simulink model "IADC_wi_SarGainError"  (Simulink 10.0)
settings: Solver=ode45  StartTime=0.0  StopTime=100e-6  RelTol=1e-3  EnableMultiTasking=on
values from neighbouring files (symbols this model uses):
  A = opgain(i)    [ExCount_wi_OPGainError_cal_m.m]    (also in ExCount_wi_OPGainError_m.m = 10000; ExCount_wi_SarGainError_cal_m.m; ExCount_wi_SarGainError_m.m; IADC_pSNDR_vs_Gain_m.m = opgain(i_opgain))
  a1 = 1/1    (= 1)    [ExCount_wi_OPGainError_cal_m.m]    (also in ExCount_wi_OPGainError_m.m; ExCount_wi_SarGainError_cal_m.m; ExCount_wi_SarGainError_m.m; IADC_pSNDR_vs_Gain_m.m)
  a11 = 1/4    (= 0.25)    [ExCount_wi_OPGainError_cal_m.m]    (also in ExCount_wi_OPGainError_m.m = 1; ExCount_wi_SarGainError_cal_m.m = 1; ExCount_wi_SarGainError_m.m = 1; IADC_pSNDR_vs_Gain_m.m = 1)
  a12 = 1    [ExCount_wi_OPGainError_cal_m.m]    (also in ExCount_wi_OPGainError_m.m; ExCount_wi_SarGainError_cal_m.m; ExCount_wi_SarGainError_m.m; IADC_pSNDR_vs_Gain_m.m)
  a2 = 1/1    (= 1)    [ExCount_wi_OPGainError_cal_m.m]    (also in ExCount_wi_OPGainError_m.m; ExCount_wi_SarGainError_cal_m.m; ExCount_wi_SarGainError_m.m; IADC_pSNDR_vs_Gain_m.m)
  A_binary = opgain_binary(i)    [ExCount_wi_OPGainError_cal_m.m]
  adder_max = vref*1    (= 0.9)    [ExCount_wi_OPGainError_cal_m.m]    (also in ExCount_wi_OPGainError_m.m; ExCount_wi_SarGainError_cal_m.m; ExCount_wi_SarGainError_m.m; IADC_pSNDR_vs_Gain_m.m)
  Amax = vref*1    (= 0.9)    [ExCount_wi_OPGainError_cal_m.m]    (also in ExCount_wi_OPGainError_m.m = 0.45; ExCount_wi_SarGainError_cal_m.m; ExCount_wi_SarGainError_m.m; IADC_pSNDR_vs_Gain_m.m = 0.45)
  b11 = 4/1    (= 4)    [ExCount_wi_OPGainError_cal_m.m]    (also in ExCount_wi_OPGainError_m.m = 1; ExCount_wi_SarGainError_cal_m.m = 1; ExCount_wi_SarGainError_m.m = 1; IADC_pSNDR_vs_Gain_m.m = 1)
  err_dac = 1.051/1000*0    (= 0)    [ExCount_wi_OPGainError_cal_m.m]
  fsig = 21.0e3    (= 21000)    [ExCount_wi_OPGainError_cal_m.m]    (also in ExCount_wi_OPGainError_m.m = 43000; ExCount_wi_SarGainError_cal_m.m; ExCount_wi_SarGainError_m.m; IADC_pSNDR_vs_Gain_m.m = 43000)
  k1 = 1/1    (= 1)    [ExCount_wi_OPGainError_cal_m.m]    (also in ExCount_wi_OPGainError_m.m; ExCount_wi_SarGainError_cal_m.m; ExCount_wi_SarGainError_m.m; IADC_pSNDR_vs_Gain_m.m)
  M = OSR-1    (= 15)    [ExCount_wi_OPGainError_cal_m.m]    (also in ExCount_wi_OPGainError_m.m; ExCount_wi_SarGainError_cal_m.m = 16; ExCount_wi_SarGainError_m.m = 16; IADC_pSNDR_vs_Gain_m.m)
  mdac = [1 1 1 1  1 1 1 1]    [ExCount_wi_OPGainError_cal_m.m]    (also in ExCount_wi_OPGainError_m.m; ExCount_wi_SarGainError_cal_m.m; ExCount_wi_SarGainError_m.m; IADC_pSNDR_vs_Gain_m.m)
  OSR = 16    [ExCount_wi_OPGainError_cal_m.m]    (also in ExCount_wi_OPGainError_m.m; ExCount_wi_SarGainError_cal_m.m; ExCount_wi_SarGainError_m.m; IADC_pSNDR_vs_Gain_m.m)
  SAR_GAIN_ERROR = SAR_GAIN_ERROR_ARR(j)    [ExCount_wi_SarGainError_cal_m.m]    (also in ExCount_wi_SarGainError_m.m)
  tclk = Ts    (= 6.25e-07)    [ExCount_wi_OPGainError_cal_m.m]    (also in ExCount_wi_OPGainError_m.m; ExCount_wi_SarGainError_cal_m.m; ExCount_wi_SarGainError_m.m; IADC_pSNDR_vs_Gain_m.m)
  vfs = vref*2    (= 1.8)    [ExCount_wi_OPGainError_cal_m.m]    (also in ExCount_wi_OPGainError_m.m; ExCount_wi_SarGainError_cal_m.m; ExCount_wi_SarGainError_m.m; IADC_pSNDR_vs_Gain_m.m)
  vin_amp = 10.^(vin_amp_dB/20)*vref    [ExCount_wi_OPGainError_cal_m.m]    (also in ExCount_wi_OPGainError_m.m = 10.^(vin_amp_db/20)*vref; ExCount_wi_SarGainError_cal_m.m = 10.^(vin_amp_dB_ARR/20)*vref; ExCount_wi_SarGainError_m.m; IADC_pSNDR_vs_Gain_m.m)
  vref = 0.9    [ExCount_wi_OPGainError_cal_m.m]    (also in ExCount_wi_OPGainError_m.m; ExCount_wi_SarGainError_cal_m.m; ExCount_wi_SarGainError_m.m; IADC_pSNDR_vs_Gain_m.m)
settings Model: LogicAnalyzerSignalOrdering=14ef830d-d328-4b55-81cf-95084106fef6  Creator=chench  LastModifiedBy=benve
settings DataIOCC: LimitDataPoints=on
settings OptimizationCC: ExpressionDepthLimit=2147483647  InitFltsAndDblsToZero=on
settings DebuggingCC: SaveWithParameterizedLinksMsg=none  SignalResolutionControl=TryResolveAllWithWarning  SolverPrmCheckMsg=warning  MultiTaskDSMMsg=warning  MultiTaskCondExecSysMsg=none  FcnCallInpInsideContextMsg=warning  AllowSymbolicDim=off  StateNameClashWarn=warning
settings GRTTargetCC: TargetFcnLib=ansi_tfl_tmw.mat  GeneratePreprocessorConditionals=Disable all
settings ConfigComp: CovExternalEMLEnable=off

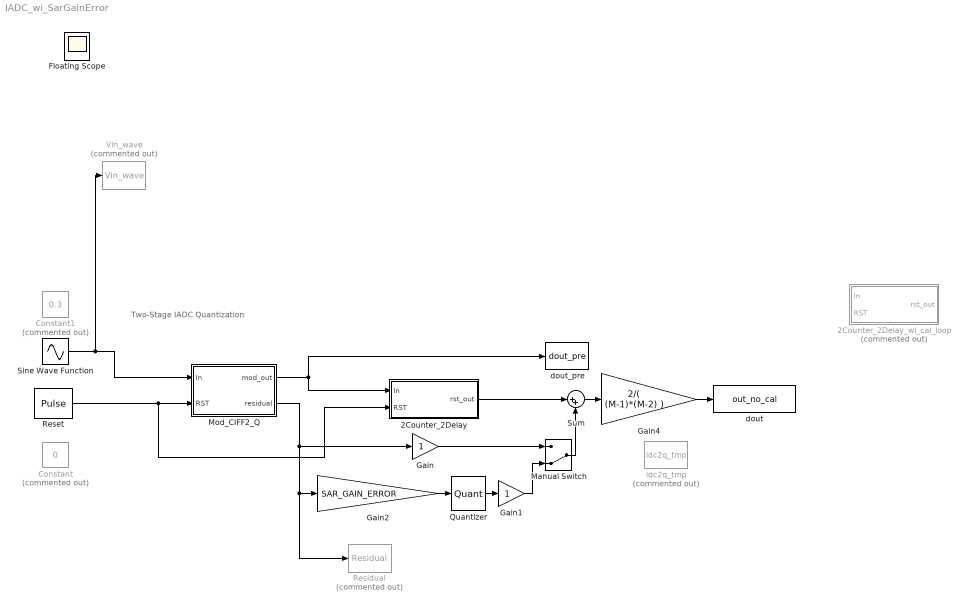
== system IADC_wi_SarGainError ==
  note: Two-Stage IADC Quantization
  2Counter_2Delay : Subsystem
  2Counter_2Delay_wi_cal_loop : Subsystem  Commented=on
  Constant : Constant  Commented=on  Value=0
  Constant1 : Constant  Commented=on  Value=0.3
  Gain : Gain
  Gain1 : Gain
  Gain2 : Gain  Gain=SAR_GAIN_ERROR
  Gain4 : Gain  Gain=2/( (M-1)*(M-2) )
  Manual Switch : ManualSwitch  CurrentSetting=0
  Mod_CIFF2_Q : Subsystem
  Quantizer : Quantizer  QuantizationInterval=vfs/1024  LinearizeAsGain=off
  Reset : DiscretePulseGenerator  Period=OSR  SampleTime=tclk
  Residual : ToWorkspace  Commented=on  VariableName=Residual  SampleTime=-1
  Sine Wave Function : Sin  Amplitude=vin_amp  Frequency=fsig*2*pi  SampleTime=tclk
  Sum : Sum  Inputs=|++
  Vin_wave : ToWorkspace  Commented=on  VariableName=Vin_wave  SampleTime=-1
  dout : ToWorkspace  VariableName=out_no_cal  SampleTime=-1
  dout_pre : ToWorkspace  VariableName=dout_pre  SampleTime=-1
  idc2q_tmp : ToWorkspace  Commented=on  VariableName=idc2q_tmp  SampleTime=-1
  Floating Scope : Scope
  wires:
  Mod_CIFF2_Q/1(mod_out) -> 2Counter_2Delay/1(In), dout_pre/1
  Gain4/1 -> dout/1
  Reset/1 -> 2Counter_2Delay/2(RST), Mod_CIFF2_Q/2(RST)
  Sum/1 -> Gain4/1
  2Counter_2Delay/1(rst_out) -> Sum/1
  Sine Wave Function/1 -> Vin_wave/1, Mod_CIFF2_Q/1(In)
  Mod_CIFF2_Q/2(residual) -> Gain/1, Gain2/1, Residual/1
  Manual Switch/1 -> Sum/2
  Gain/1 -> Manual Switch/1
  Quantizer/1 -> Gain1/1
  Gain1/1 -> Manual Switch/2
  Gain2/1 -> Quantizer/1

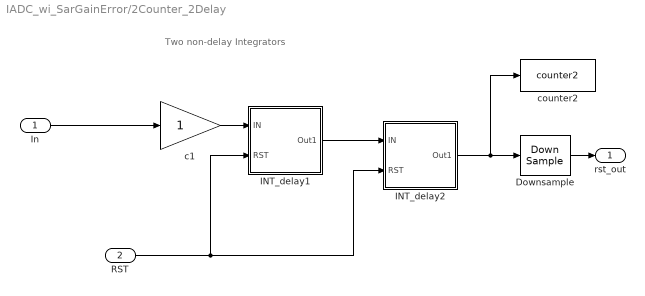
== system IADC_wi_SarGainError/2Counter_2Delay ==
  note: Two non-delay Integrators
  In : Inport
  RST : Inport  Port=2
  Downsample : DownSample  N=OSR  phase=OSR-1  RateOptions=Allow multirate processing
  INT_delay1 : Subsystem
  INT_delay2 : Subsystem
  c1 : Gain  SaturateOnIntegerOverflow=on  OutDataTypeStr=Inherit: Same as input  ParamDataTypeStr=Inherit: Same as input
  counter2 : ToWorkspace  VariableName=counter2  SampleTime=-1
  rst_out : Outport  VectorParamsAs1DForOutWhenUnconnected=off
  wires:
  INT_delay1/1(Out1) -> INT_delay2/1(IN)
  c1/1 -> INT_delay1/1(IN)
  INT_delay2/1(Out1) -> Downsample/1, counter2/1
  RST/1 -> INT_delay1/2(RST), INT_delay2/2(RST)
  Downsample/1 -> rst_out/1
  In/1 -> c1/1

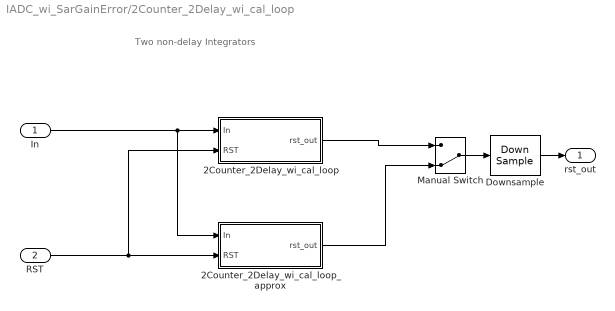
== system IADC_wi_SarGainError/2Counter_2Delay_wi_cal_loop ==
  note: Two non-delay Integrators
  In : Inport
  RST : Inport  Port=2
  2Counter_2Delay_wi_cal_loop : Subsystem
  2Counter_2Delay_wi_cal_loop_approx : Subsystem
  Downsample : DownSample  N=OSR  phase=OSR-1  RateOptions=Allow multirate processing
  Manual Switch : ManualSwitch  CurrentSetting=0
  rst_out : Outport  VectorParamsAs1DForOutWhenUnconnected=off
  wires:
  Downsample/1 -> rst_out/1
  In/1 -> 2Counter_2Delay_wi_cal_loop_approx/1(In), 2Counter_2Delay_wi_cal_loop/1(In)
  RST/1 -> 2Counter_2Delay_wi_cal_loop/2(RST), 2Counter_2Delay_wi_cal_loop_approx/2(RST)
  Manual Switch/1 -> Downsample/1
  2Counter_2Delay_wi_cal_loop/1(rst_out) -> Manual Switch/1
  2Counter_2Delay_wi_cal_loop_approx/1(rst_out) -> Manual Switch/2

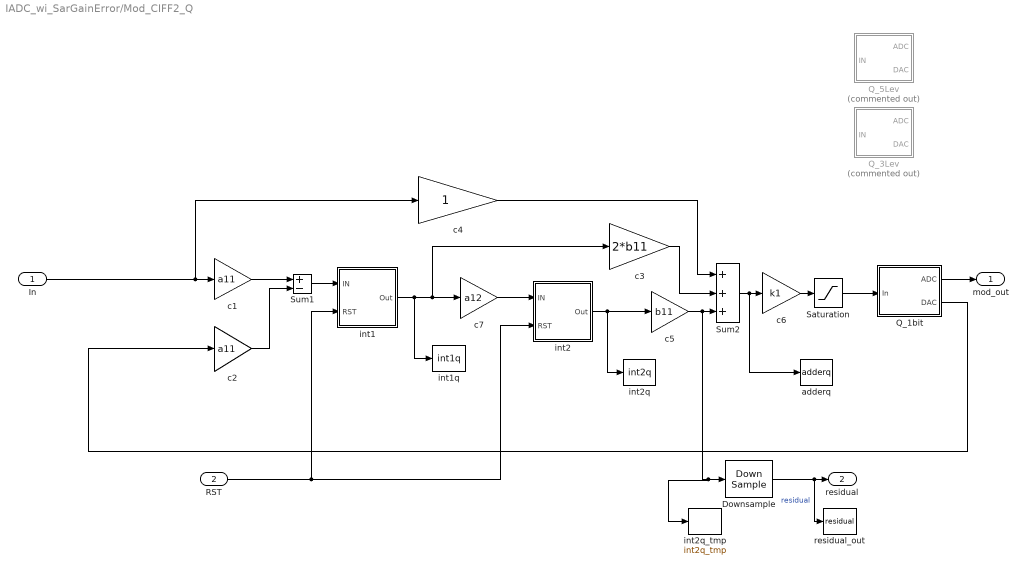
== system IADC_wi_SarGainError/Mod_CIFF2_Q ==
  In : Inport
  RST : Inport  Port=2
  Downsample : DownSample  N=OSR  phase=OSR-1  RateOptions=Allow multirate processing
  Q_1bit : Subsystem
  Q_3Lev : Subsystem  Commented=on
  Q_5Lev : Subsystem  Commented=on
  Saturation : Saturate  UpperLimit=adder_max*1  LowerLimit=-1*adder_max
  Sum1 : Sum  Inputs=+-  SaturateOnIntegerOverflow=on  InputSameDT=on  OutDataTypeStr=Inherit: Same as first input
  Sum2 : Sum  Inputs=+++  SaturateOnIntegerOverflow=on  InputSameDT=on  OutDataTypeStr=Inherit: Same as first input
  adderq : ToWorkspace  VariableName=adderq  SampleTime=-1
  c1 : Gain  Gain=a11  SaturateOnIntegerOverflow=on  OutDataTypeStr=Inherit: Same as input  ParamDataTypeStr=Inherit: Same as input
  c2 : Gain  Gain=a11  SaturateOnIntegerOverflow=on  OutDataTypeStr=Inherit: Same as input  ParamDataTypeStr=Inherit: Same as input
  c3 : Gain  Gain=2*b11  SaturateOnIntegerOverflow=on  OutDataTypeStr=Inherit: Same as input  ParamDataTypeStr=Inherit: Same as input
  c4 : Gain  SaturateOnIntegerOverflow=on  OutDataTypeStr=Inherit: Same as input  ParamDataTypeStr=Inherit: Same as input
  c5 : Gain  Gain=b11  SaturateOnIntegerOverflow=on  OutDataTypeStr=Inherit: Same as input  ParamDataTypeStr=Inherit: Same as input
  c6 : Gain  Gain=k1  SaturateOnIntegerOverflow=on  OutDataTypeStr=Inherit: Same as input  ParamDataTypeStr=Inherit: Same as input
  c7 : Gain  Gain=a12  SaturateOnIntegerOverflow=on  OutDataTypeStr=Inherit: Same as input  ParamDataTypeStr=Inherit: Same as input
  int1 : Subsystem
  int1q : ToWorkspace  VariableName=int1q  SampleTime=-1
  int2 : Subsystem
  int2q : ToWorkspace  VariableName=int2q  SampleTime=-1
  int2q_tmp : ToWorkspace  VariableName=int2q_tmp  SampleTime=-1
  residual_out : ToWorkspace  VariableName=residual  SampleTime=-1
  mod_out : Outport  VectorParamsAs1DForOutWhenUnconnected=off
  residual : Outport  Port=2  VectorParamsAs1DForOutWhenUnconnected=off
  wires:
  int1/1(Out) -> int1q/1, c7/1, c3/1
  int2/1(Out) -> c5/1, int2q/1
  c3/1 -> Sum2/2
  Saturation/1 -> Q_1bit/1(In)
  c5/1 -> int2q_tmp/1, Downsample/1, Sum2/3
  Q_1bit/1(ADC) -> mod_out/1
  c1/1 -> Sum1/1
  c2/1 -> Sum1/2
  In/1 -> c1/1, c4/1
  Sum1/1 -> int1/1(IN)
  c4/1 -> Sum2/1
  c6/1 -> Saturation/1
  Sum2/1 -> adderq/1, c6/1
  Q_1bit/2(DAC) -> c2/1
  Downsample/1 -> residual_out/1, residual/1  "residual"
  c7/1 -> int2/1(IN)
  RST/1 -> int2/2(RST), int1/2(RST)

== system IADC_wi_SarGainError/2Counter_2Delay/INT_delay1 ==
  IN : Inport
  RST : Inport  Port=2
  Delay1 : Delay  DelayLength=1  InitialCondition=0  ExternalReset=Rising
      settings: InputPortMap=u0,r5
  Sum : Sum  SaturateOnIntegerOverflow=on  InputSameDT=on  OutDataTypeStr=Inherit: Same as first input
  Out1 : Outport  VectorParamsAs1DForOutWhenUnconnected=off
  wires:
  IN/1 -> Sum/1
  Delay1/1 -> Sum/2, Out1/1
  RST/1 -> Delay1/2
  Sum/1 -> Delay1/1

== system IADC_wi_SarGainError/2Counter_2Delay/INT_delay2 ==
  IN : Inport
  RST : Inport  Port=2
  Delay1 : Delay  DelayLength=1  InitialCondition=0  ExternalReset=Rising
      settings: InputPortMap=u0,r5
  Sum : Sum  SaturateOnIntegerOverflow=on  InputSameDT=on  OutDataTypeStr=Inherit: Same as first input
  Out1 : Outport  VectorParamsAs1DForOutWhenUnconnected=off
  wires:
  IN/1 -> Sum/1
  Delay1/1 -> Sum/2, Out1/1
  RST/1 -> Delay1/2
  Sum/1 -> Delay1/1

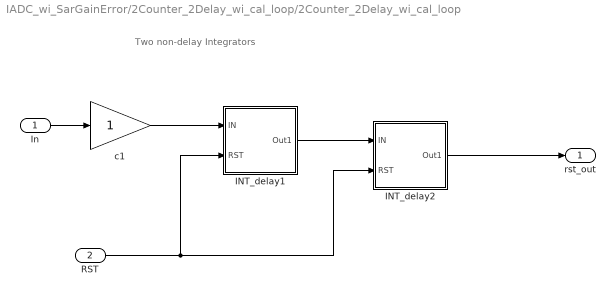
== system IADC_wi_SarGainError/2Counter_2Delay_wi_cal_loop/2Counter_2Delay_wi_cal_loop ==
  note: Two non-delay Integrators
  In : Inport
  RST : Inport  Port=2
  INT_delay1 : Subsystem
  INT_delay2 : Subsystem
  c1 : Gain  SaturateOnIntegerOverflow=on  OutDataTypeStr=Inherit: Same as input  ParamDataTypeStr=Inherit: Same as input
  rst_out : Outport  VectorParamsAs1DForOutWhenUnconnected=off
  wires:
  RST/1 -> INT_delay1/2(RST), INT_delay2/2(RST)
  INT_delay2/1(Out1) -> rst_out/1
  In/1 -> c1/1
  c1/1 -> INT_delay1/1(IN)
  INT_delay1/1(Out1) -> INT_delay2/1(IN)

== system IADC_wi_SarGainError/2Counter_2Delay_wi_cal_loop/2Counter_2Delay_wi_cal_loop_approx ==
  note: Two non-delay Integrators
  In : Inport
  RST : Inport  Port=2
  INT_delay1 : Subsystem
  INT_delay2 : Subsystem
  c1 : Gain  SaturateOnIntegerOverflow=on  OutDataTypeStr=Inherit: Same as input  ParamDataTypeStr=Inherit: Same as input
  rst_out : Outport  VectorParamsAs1DForOutWhenUnconnected=off
  wires:
  RST/1 -> INT_delay1/2(RST), INT_delay2/2(RST)
  INT_delay2/1(Out1) -> rst_out/1
  In/1 -> c1/1
  c1/1 -> INT_delay1/1(IN)
  INT_delay1/1(Out1) -> INT_delay2/1(IN)

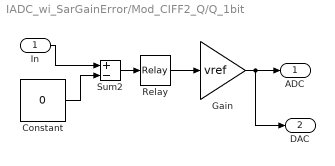
== system IADC_wi_SarGainError/Mod_CIFF2_Q/Q_1bit ==
  In : Inport
  Constant : Constant  Value=0
  Gain : Gain  Gain=vref
  Relay : Relay  OffOutputValue=-1  SampleTime=tclk
  Sum2 : Sum  Inputs=+-  SaturateOnIntegerOverflow=on  InputSameDT=on  OutDataTypeStr=Inherit: Same as first input
  ADC : Outport  VectorParamsAs1DForOutWhenUnconnected=off
  DAC : Outport  Port=2  VectorParamsAs1DForOutWhenUnconnected=off
  wires:
  Sum2/1 -> Relay/1
  Constant/1 -> Sum2/2
  In/1 -> Sum2/1
  Relay/1 -> Gain/1
  Gain/1 -> ADC/1, DAC/1

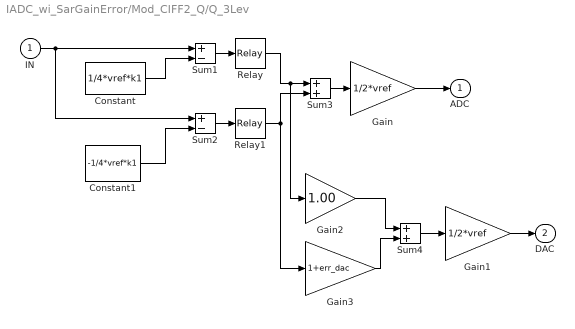
== system IADC_wi_SarGainError/Mod_CIFF2_Q/Q_3Lev ==
  IN : Inport
  Constant : Constant  Value=1/4*vref*k1
  Constant1 : Constant  Value=-1/4*vref*k1
  Gain : Gain  Gain=1/2*vref
  Gain1 : Gain  Gain=1/2*vref
  Gain2 : Gain  Gain=1.00
  Gain3 : Gain  Gain=1+err_dac
  Relay : Relay  OffOutputValue=-1  SampleTime=tclk
  Relay1 : Relay  OffOutputValue=-1  SampleTime=tclk
  Sum1 : Sum  Inputs=+-  SaturateOnIntegerOverflow=on  InputSameDT=on  OutDataTypeStr=Inherit: Same as first input
  Sum2 : Sum  Inputs=+-  SaturateOnIntegerOverflow=on  InputSameDT=on  OutDataTypeStr=Inherit: Same as first input
  Sum3 : Sum  SaturateOnIntegerOverflow=on  InputSameDT=on  OutDataTypeStr=Inherit: Same as first input
  Sum4 : Sum  SaturateOnIntegerOverflow=on  InputSameDT=on  OutDataTypeStr=Inherit: Same as first input
  ADC : Outport  VectorParamsAs1DForOutWhenUnconnected=off
  DAC : Outport  Port=2  VectorParamsAs1DForOutWhenUnconnected=off
  wires:
  Sum1/1 -> Relay/1
  Sum2/1 -> Relay1/1
  IN/1 -> Sum1/1, Sum2/1
  Constant/1 -> Sum1/2
  Constant1/1 -> Sum2/2
  Relay/1 -> Sum3/1, Gain2/1
  Relay1/1 -> Sum3/2, Gain3/1
  Sum3/1 -> Gain/1
  Gain/1 -> ADC/1
  Sum4/1 -> Gain1/1
  Gain2/1 -> Sum4/1
  Gain1/1 -> DAC/1
  Gain3/1 -> Sum4/2

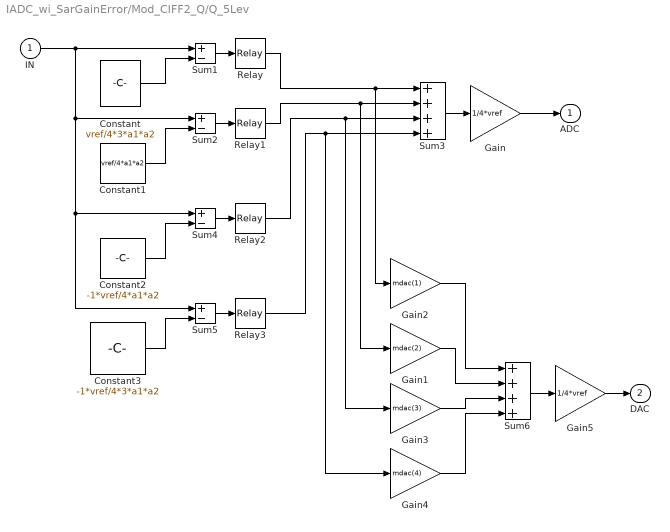
== system IADC_wi_SarGainError/Mod_CIFF2_Q/Q_5Lev ==
  IN : Inport
  Constant : Constant  Value=vref/4*3*a1*a2
  Constant1 : Constant  Value=vref/4*a1*a2
  Constant2 : Constant  Value=-1*vref/4*a1*a2
  Constant3 : Constant  Value=-1*vref/4*3*a1*a2
  Gain : Gain  Gain=1/4*vref
  Gain1 : Gain  Gain=mdac(2)
  Gain2 : Gain  Gain=mdac(1)
  Gain3 : Gain  Gain=mdac(3)
  Gain4 : Gain  Gain=mdac(4)
  Gain5 : Gain  Gain=1/4*vref
  Relay{,1..3} (4 alike) : Relay  OffOutputValue=-1  SampleTime=tclk
  Sum{1..2,4..5} (4 alike) : Sum  Inputs=+-  SaturateOnIntegerOverflow=on  InputSameDT=on  OutDataTypeStr=Inherit: Same as first input
  Sum3 : Sum  Inputs=++++  SaturateOnIntegerOverflow=on  InputSameDT=on  OutDataTypeStr=Inherit: Same as first input
  Sum6 : Sum  Inputs=++++  SaturateOnIntegerOverflow=on  InputSameDT=on  OutDataTypeStr=Inherit: Same as first input
  ADC : Outport  VectorParamsAs1DForOutWhenUnconnected=off
  DAC : Outport  Port=2  VectorParamsAs1DForOutWhenUnconnected=off
  wires:
  Sum1/1 -> Relay/1
  Sum2/1 -> Relay1/1
  IN/1 -> Sum1/1, Sum2/1, Sum4/1, Sum5/1
  Constant/1 -> Sum1/2
  Constant1/1 -> Sum2/2
  Relay/1 -> Sum3/1, Gain2/1
  Relay1/1 -> Sum3/2, Gain1/1
  Sum3/1 -> Gain/1
  Gain/1 -> ADC/1
  Sum4/1 -> Relay2/1
  Constant2/1 -> Sum4/2
  Relay2/1 -> Sum3/3, Gain3/1
  Sum5/1 -> Relay3/1
  Constant3/1 -> Sum5/2
  Relay3/1 -> Sum3/4, Gain4/1
  Gain2/1 -> Sum6/1
  Gain1/1 -> Sum6/2
  Gain3/1 -> Sum6/3
  Gain4/1 -> Sum6/4
  Sum6/1 -> Gain5/1
  Gain5/1 -> DAC/1

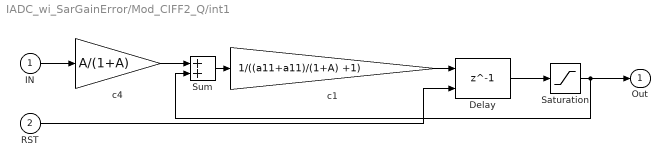
== system IADC_wi_SarGainError/Mod_CIFF2_Q/int1 ==
  IN : Inport
  RST : Inport  Port=2
  Delay : Delay  DelayLength=1  InitialCondition=0  ExternalReset=Rising
      settings: InputPortMap=u0,r5
  Saturation : Saturate  UpperLimit=Amax  LowerLimit=-1*Amax
  Sum : Sum  SaturateOnIntegerOverflow=on  InputSameDT=on  OutDataTypeStr=Inherit: Same as first input
  c1 : Gain  Gain=1/((a11+a11)/(1+A) +1)  SaturateOnIntegerOverflow=on  OutDataTypeStr=Inherit: Same as input  ParamDataTypeStr=Inherit: Same as input
  c4 : Gain  Gain=A/(1+A)  SaturateOnIntegerOverflow=on  OutDataTypeStr=Inherit: Same as input  ParamDataTypeStr=Inherit: Same as input
  Out : Outport  VectorParamsAs1DForOutWhenUnconnected=off
  wires:
  Delay/1 -> Saturation/1
  IN/1 -> c4/1
  Saturation/1 -> Sum/2, Out/1
  RST/1 -> Delay/2
  c4/1 -> Sum/1
  Sum/1 -> c1/1
  c1/1 -> Delay/1

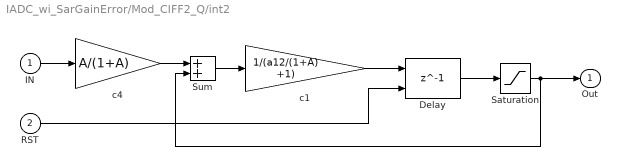
== system IADC_wi_SarGainError/Mod_CIFF2_Q/int2 ==
  IN : Inport
  RST : Inport  Port=2
  Delay : Delay  DelayLength=1  InitialCondition=0  ExternalReset=Rising
      settings: InputPortMap=u0,r5
  Saturation : Saturate  UpperLimit=Amax  LowerLimit=-1*Amax
  Sum : Sum  SaturateOnIntegerOverflow=on  InputSameDT=on  OutDataTypeStr=Inherit: Same as first input
  c1 : Gain  Gain=1/(a12/(1+A) +1)  SaturateOnIntegerOverflow=on  OutDataTypeStr=Inherit: Same as input  ParamDataTypeStr=Inherit: Same as input
  c4 : Gain  Gain=A/(1+A)  SaturateOnIntegerOverflow=on  OutDataTypeStr=Inherit: Same as input  ParamDataTypeStr=Inherit: Same as input
  Out : Outport  VectorParamsAs1DForOutWhenUnconnected=off
  wires:
  Delay/1 -> Saturation/1
  IN/1 -> c4/1
  Saturation/1 -> Sum/2, Out/1
  RST/1 -> Delay/2
  c4/1 -> Sum/1
  Sum/1 -> c1/1
  c1/1 -> Delay/1

== system IADC_wi_SarGainError/2Counter_2Delay_wi_cal_loop/2Counter_2Delay_wi_cal_loop/INT_delay1 ==
  IN : Inport
  RST : Inport  Port=2
  Delay1 : Delay  DelayLength=1  InitialCondition=0  ExternalReset=Rising
      settings: InputPortMap=u0,r5
  Sum : Sum  SaturateOnIntegerOverflow=on  InputSameDT=on  OutDataTypeStr=Inherit: Same as first input
  c1 : Gain  Gain=1/((a11+a11)/(1+A) +1)  SaturateOnIntegerOverflow=on  OutDataTypeStr=Inherit: Same as input  ParamDataTypeStr=Inherit: Same as input
  Out1 : Outport  VectorParamsAs1DForOutWhenUnconnected=off
  wires:
  IN/1 -> Sum/1
  Delay1/1 -> Sum/2, Out1/1
  RST/1 -> Delay1/2
  c1/1 -> Delay1/1
  Sum/1 -> c1/1

== system IADC_wi_SarGainError/2Counter_2Delay_wi_cal_loop/2Counter_2Delay_wi_cal_loop/INT_delay2 ==
  IN : Inport
  RST : Inport  Port=2
  Delay1 : Delay  DelayLength=1  InitialCondition=0  ExternalReset=Rising
      settings: InputPortMap=u0,r5
  Sum : Sum  SaturateOnIntegerOverflow=on  InputSameDT=on  OutDataTypeStr=Inherit: Same as first input
  c1 : Gain  Gain=1/(a12/(1+A) +1)  SaturateOnIntegerOverflow=on  OutDataTypeStr=Inherit: Same as input  ParamDataTypeStr=Inherit: Same as input
  Out1 : Outport  VectorParamsAs1DForOutWhenUnconnected=off
  wires:
  IN/1 -> Sum/1
  Delay1/1 -> Sum/2, Out1/1
  RST/1 -> Delay1/2
  c1/1 -> Delay1/1
  Sum/1 -> c1/1

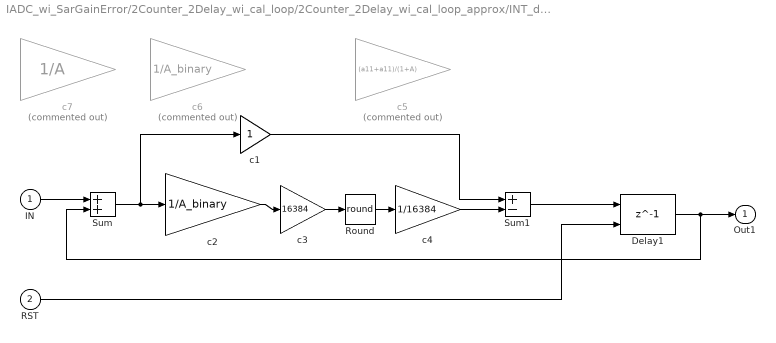
== system IADC_wi_SarGainError/2Counter_2Delay_wi_cal_loop/2Counter_2Delay_wi_cal_loop_approx/INT_delay1 ==
  IN : Inport
  RST : Inport  Port=2
  Delay1 : Delay  DelayLength=1  InitialCondition=0  ExternalReset=Rising
      settings: InputPortMap=u0,r5
  Round : Rounding  Operator=round
  Sum : Sum  SaturateOnIntegerOverflow=on  InputSameDT=on  OutDataTypeStr=Inherit: Same as first input
  Sum1 : Sum  Inputs=+-  SaturateOnIntegerOverflow=on  InputSameDT=on  OutDataTypeStr=Inherit: Same as first input
  c1 : Gain  SaturateOnIntegerOverflow=on  OutDataTypeStr=Inherit: Same as input  ParamDataTypeStr=Inherit: Same as input
  c2 : Gain  Gain=1/A_binary  SaturateOnIntegerOverflow=on  OutDataTypeStr=Inherit: Same as input  ParamDataTypeStr=Inherit: Same as input
  c3 : Gain  Gain=16384  SaturateOnIntegerOverflow=on  OutDataTypeStr=Inherit: Same as input  ParamDataTypeStr=Inherit: Same as input
  c4 : Gain  Gain=1/16384  SaturateOnIntegerOverflow=on  OutDataTypeStr=Inherit: Same as input  ParamDataTypeStr=Inherit: Same as input
  c5 : Gain  Commented=on  Gain=(a11+a11)/(1+A)  SaturateOnIntegerOverflow=on  OutDataTypeStr=Inherit: Same as input  ParamDataTypeStr=Inherit: Same as input
  c6 : Gain  Commented=on  Gain=1/A_binary  SaturateOnIntegerOverflow=on  OutDataTypeStr=Inherit: Same as input  ParamDataTypeStr=Inherit: Same as input
  c7 : Gain  Commented=on  Gain=1/A  SaturateOnIntegerOverflow=on  OutDataTypeStr=Inherit: Same as input  ParamDataTypeStr=Inherit: Same as input
  Out1 : Outport  VectorParamsAs1DForOutWhenUnconnected=off
  wires:
  IN/1 -> Sum/1
  Delay1/1 -> Sum/2, Out1/1
  RST/1 -> Delay1/2
  Sum/1 -> c2/1, c1/1
  c1/1 -> Sum1/1
  Sum1/1 -> Delay1/1
  c2/1 -> c3/1
  c3/1 -> Round/1
  Round/1 -> c4/1
  c4/1 -> Sum1/2

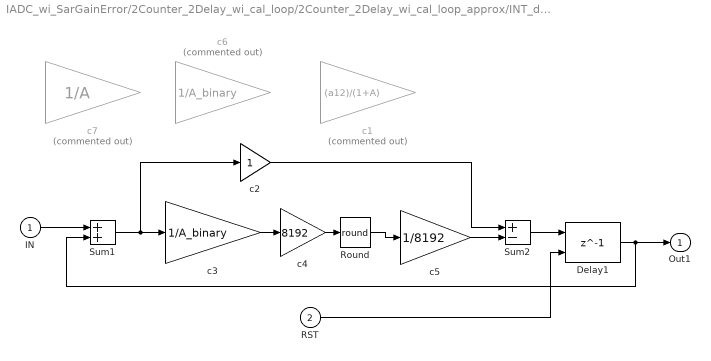
== system IADC_wi_SarGainError/2Counter_2Delay_wi_cal_loop/2Counter_2Delay_wi_cal_loop_approx/INT_delay2 ==
  IN : Inport
  RST : Inport  Port=2
  Delay1 : Delay  DelayLength=1  InitialCondition=0  ExternalReset=Rising
      settings: InputPortMap=u0,r5
  Round : Rounding  Operator=round
  Sum1 : Sum  SaturateOnIntegerOverflow=on  InputSameDT=on  OutDataTypeStr=Inherit: Same as first input
  Sum2 : Sum  Inputs=+-  SaturateOnIntegerOverflow=on  InputSameDT=on  OutDataTypeStr=Inherit: Same as first input
  c1 : Gain  Commented=on  Gain=(a12)/(1+A)  SaturateOnIntegerOverflow=on  OutDataTypeStr=Inherit: Same as input  ParamDataTypeStr=Inherit: Same as input
  c2 : Gain  SaturateOnIntegerOverflow=on  OutDataTypeStr=Inherit: Same as input  ParamDataTypeStr=Inherit: Same as input
  c3 : Gain  Gain=1/A_binary  SaturateOnIntegerOverflow=on  OutDataTypeStr=Inherit: Same as input  ParamDataTypeStr=Inherit: Same as input
  c4 : Gain  Gain=8192  SaturateOnIntegerOverflow=on  OutDataTypeStr=Inherit: Same as input  ParamDataTypeStr=Inherit: Same as input
  c5 : Gain  Gain=1/8192  SaturateOnIntegerOverflow=on  OutDataTypeStr=Inherit: Same as input  ParamDataTypeStr=Inherit: Same as input
  c6 : Gain  Commented=on  Gain=1/A_binary  SaturateOnIntegerOverflow=on  OutDataTypeStr=Inherit: Same as input  ParamDataTypeStr=Inherit: Same as input
  c7 : Gain  Commented=on  Gain=1/A  SaturateOnIntegerOverflow=on  OutDataTypeStr=Inherit: Same as input  ParamDataTypeStr=Inherit: Same as input
  Out1 : Outport  VectorParamsAs1DForOutWhenUnconnected=off
  wires:
  IN/1 -> Sum1/1
  Delay1/1 -> Sum1/2, Out1/1
  RST/1 -> Delay1/2
  Sum2/1 -> Delay1/1
  Round/1 -> c5/1
  c4/1 -> Round/1
  Sum1/1 -> c3/1, c2/1
  c2/1 -> Sum2/1
  c3/1 -> c4/1
  c5/1 -> Sum2/2
